simulink model "tau_11_1"  (R2019b)
settings: Solver=VariableStepAuto  StartTime=0.0  StopTime=1  RelTol=1e-3
libraries: simulink x16, slctrlblks x1
settings Model: PacingRate=0.001800  Creator=Sergey  LastModifiedBy=Sergey

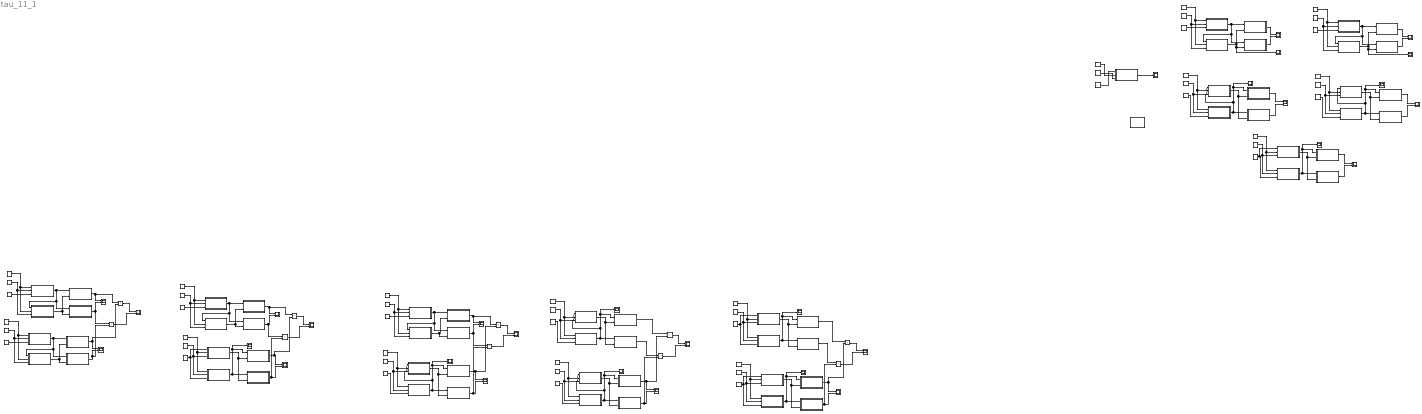
== system tau_11_1 ==
  note: А-ЗВЕНО
  note: П-ЗВЕНО
  note: РИ-ЗВЕНО
  note: ИИ-ЗВЕНО
  note: РД-ЗВЕНО
  note: А-ЗВЕНО
  note: А-ЗВЕНО
  note: А-ЗВЕНО
  note: РД-ЗВЕНО
  note: А-ЗВЕНО
  note: РИ-ЗВЕНО
  note: РИ-ЗВЕНО
  note: РИ-ЗВЕНО
  note: РД-ЗВЕНО
  note: РД-ЗВЕНО
  Bode Plot : slctrlblks/Model Verification/Check Bode  Characteristics  InstantiateOnLoad=on  SaveOperatingPoints=off  LinearizationIOs={}  LinearizeAt=SnapshotTimes  SnapshotTimes=[0]  TriggerType=rising  SampleTime=auto  RateConversionMethod=zoh  PreWarpFreq=10  UseExactDelayModel=off  UseFullBlockNameLabels=off  UseBusSignalLabels=off  enabled=on  stopWhenAssertionFail=off  export=off  ViewDlgPos=[1 41 1920 963]  OpenViewOnLoad=off  LaunchViewOnOpen=off  FrequencyUnits=rad/s  MagnitudeUnits=dB  PhaseUnits=deg  TimeUnits=seconds  EnableUpperBound=off  UpperBoundFrequencies=[]  UpperBoundMagnitudes=[]  EnableLowerBound=off  LowerBoundFrequencies=[]  LowerBoundMagnitudes=[]
      settings: SourceProductName=Simulink Control Design
  Constant{,4,8,10,12,14,16,18,20,22,24,26,28,30} (14 alike) : Constant  Value=0.5
  Constant{1,3,5,7,9,11,13,15,17,19,21,23,25,27,29,31} (16 alike) : Constant  Value=9
  Constant2 : Constant  Value=0
  Constant6 : Constant  Value=0
  MATLAB Function : MATLAB Function  TreatAsAtomicUnit=on
  MATLAB Function1 : MATLAB Function  TreatAsAtomicUnit=on
  MATLAB Function10 : MATLAB Function  TreatAsAtomicUnit=on
  MATLAB Function11 : MATLAB Function  TreatAsAtomicUnit=on
  MATLAB Function12 : MATLAB Function  TreatAsAtomicUnit=on
  MATLAB Function13 : MATLAB Function  TreatAsAtomicUnit=on
  MATLAB Function14 : MATLAB Function  TreatAsAtomicUnit=on
  MATLAB Function15 : MATLAB Function  TreatAsAtomicUnit=on
  MATLAB Function16 : MATLAB Function  TreatAsAtomicUnit=on
  MATLAB Function17 : MATLAB Function  TreatAsAtomicUnit=on
  MATLAB Function18 : MATLAB Function  TreatAsAtomicUnit=on
  MATLAB Function19 : MATLAB Function  TreatAsAtomicUnit=on
  MATLAB Function2 : MATLAB Function  TreatAsAtomicUnit=on
  MATLAB Function20 : MATLAB Function  TreatAsAtomicUnit=on
  MATLAB Function21 : MATLAB Function  TreatAsAtomicUnit=on
  MATLAB Function22 : MATLAB Function  TreatAsAtomicUnit=on
  MATLAB Function23 : MATLAB Function  TreatAsAtomicUnit=on
  MATLAB Function24 : MATLAB Function  TreatAsAtomicUnit=on
  MATLAB Function25 : MATLAB Function  TreatAsAtomicUnit=on
  MATLAB Function26 : MATLAB Function  TreatAsAtomicUnit=on
  MATLAB Function27 : MATLAB Function  TreatAsAtomicUnit=on
  MATLAB Function28 : MATLAB Function  TreatAsAtomicUnit=on
  MATLAB Function29 : MATLAB Function  TreatAsAtomicUnit=on
  MATLAB Function3 : MATLAB Function  TreatAsAtomicUnit=on
  MATLAB Function30 : MATLAB Function  TreatAsAtomicUnit=on
  MATLAB Function31 : MATLAB Function  TreatAsAtomicUnit=on
  MATLAB Function32 : MATLAB Function  TreatAsAtomicUnit=on
  MATLAB Function33 : MATLAB Function  TreatAsAtomicUnit=on
  MATLAB Function34 : MATLAB Function  TreatAsAtomicUnit=on
  MATLAB Function35 : MATLAB Function  TreatAsAtomicUnit=on
  MATLAB Function36 : MATLAB Function  TreatAsAtomicUnit=on
  MATLAB Function37 : MATLAB Function  TreatAsAtomicUnit=on
  MATLAB Function38 : MATLAB Function  TreatAsAtomicUnit=on
  MATLAB Function39 : MATLAB Function  TreatAsAtomicUnit=on
  MATLAB Function4 : MATLAB Function  TreatAsAtomicUnit=on
  MATLAB Function40 : MATLAB Function  TreatAsAtomicUnit=on
  MATLAB Function41 : MATLAB Function  TreatAsAtomicUnit=on
  MATLAB Function42 : MATLAB Function  TreatAsAtomicUnit=on
  MATLAB Function43 : MATLAB Function  TreatAsAtomicUnit=on
  MATLAB Function44 : MATLAB Function  TreatAsAtomicUnit=on
  MATLAB Function45 : MATLAB Function  TreatAsAtomicUnit=on
  MATLAB Function46 : MATLAB Function  TreatAsAtomicUnit=on
  MATLAB Function47 : MATLAB Function  TreatAsAtomicUnit=on
  MATLAB Function48 : MATLAB Function  TreatAsAtomicUnit=on
  MATLAB Function49 : MATLAB Function  TreatAsAtomicUnit=on
  MATLAB Function5 : MATLAB Function  TreatAsAtomicUnit=on
  MATLAB Function50 : MATLAB Function  TreatAsAtomicUnit=on
  MATLAB Function51 : MATLAB Function  TreatAsAtomicUnit=on
  MATLAB Function52 : MATLAB Function  TreatAsAtomicUnit=on
  MATLAB Function53 : MATLAB Function  TreatAsAtomicUnit=on
  MATLAB Function54 : MATLAB Function  TreatAsAtomicUnit=on
  MATLAB Function55 : MATLAB Function  TreatAsAtomicUnit=on
  MATLAB Function56 : MATLAB Function  TreatAsAtomicUnit=on
  MATLAB Function57 : MATLAB Function  TreatAsAtomicUnit=on
  MATLAB Function58 : MATLAB Function  TreatAsAtomicUnit=on
  MATLAB Function59 : MATLAB Function  TreatAsAtomicUnit=on
  MATLAB Function6 : MATLAB Function  TreatAsAtomicUnit=on
  MATLAB Function60 : MATLAB Function  TreatAsAtomicUnit=on
  MATLAB Function7 : MATLAB Function  TreatAsAtomicUnit=on
  MATLAB Function8 : MATLAB Function  TreatAsAtomicUnit=on
  MATLAB Function9 : MATLAB Function  TreatAsAtomicUnit=on
  Product{,1..9} (10 alike) : Product
  Ramp{,1..4,6..15} (15 alike) : simulink/Sources/Ramp  slope=1  start=0  InitialOutput=0
  Ramp5 : simulink/Sources/Ramp  slope=.0001  start=0  InitialOutput=0
  Scope{,2,4,6,8,11..17,19,21..22,25..26,28} (18 alike) : Scope  NumInputPorts=2
  Scope{1,3,5,7,9..10,18,20,23..24,27,29} (12 alike) : Scope
  wires:
  Ramp/1 -> MATLAB Function1/2(w), MATLAB Function/1(w)
  Constant/1 -> MATLAB Function1/3(T), MATLAB Function/2(T)
  Constant1/1 -> MATLAB Function/3(k)
  MATLAB Function/1(R) -> MATLAB Function3/1(R), MATLAB Function1/1(R), MATLAB Function2/1(R)
  MATLAB Function1/1(I) -> Scope1/1, MATLAB Function3/2(I), MATLAB Function2/2(I)
  MATLAB Function2/1(A) -> Scope/1
  MATLAB Function3/1(fi) -> Scope/2
  MATLAB Function7/1(fi) -> Scope2/2
  MATLAB Function6/1(A) -> Scope2/1
  MATLAB Function5/1(I) -> MATLAB Function6/2(I), MATLAB Function7/2(I), Scope3/1
  MATLAB Function4/1(R) -> MATLAB Function6/1(R), MATLAB Function5/1(R), MATLAB Function7/1(R)
  Constant3/1 -> MATLAB Function4/3(k)
  Constant2/1 -> MATLAB Function4/2(T), MATLAB Function5/3(T)
  Ramp1/1 -> MATLAB Function4/1(w), MATLAB Function5/2(w)
  MATLAB Function11/1(fi) -> Scope4/2
  MATLAB Function10/1(A) -> Scope4/1
  MATLAB Function9/1(R) -> MATLAB Function11/2(R), MATLAB Function10/2(R)
  MATLAB Function8/1(I) -> Scope5/1, MATLAB Function10/1(I), MATLAB Function9/3(I), MATLAB Function11/1(I)
  Constant5/1 -> MATLAB Function8/3(k)
  Constant4/1 -> MATLAB Function8/2(T), MATLAB Function9/2(T)
  Ramp2/1 -> MATLAB Function8/1(w), MATLAB Function9/1(w)
  Ramp3/1 -> MATLAB Function15/2(w), MATLAB Function14/1(w)
  Constant6/1 -> MATLAB Function15/3(T), MATLAB Function14/2(T)
  Constant7/1 -> MATLAB Function14/3(k)
  MATLAB Function14/1(I) -> MATLAB Function13/1(I), MATLAB Function15/1(I), MATLAB Function12/1(I), Scope7/1
  MATLAB Function15/1(R) -> MATLAB Function12/2(R), MATLAB Function13/2(R)
  MATLAB Function12/1(A) -> Scope6/1
  MATLAB Function13/1(fi) -> Scope6/2
  Ramp4/1 -> MATLAB Function19/2(w), MATLAB Function18/1(w)
  Constant8/1 -> MATLAB Function19/3(T), MATLAB Function18/2(T)
  Constant9/1 -> MATLAB Function19/1(k), MATLAB Function18/3(k)
  MATLAB Function18/1(I) -> MATLAB Function17/1(I), MATLAB Function16/1(I), Scope9/1
  MATLAB Function19/1(R) -> MATLAB Function16/2(R), MATLAB Function17/2(R)
  MATLAB Function16/1(A) -> Scope8/1
  MATLAB Function17/1(fi) -> Scope8/2
  Constant11/1 -> MATLAB Function20/1(k)
  Constant10/1 -> MATLAB Function20/3(T)
  MATLAB Function20/1(R) -> Scope10/1
  Ramp5/1 -> MATLAB Function20/2(w)
  MATLAB Function24/1(fi) -> Product/1, Scope11/2
  MATLAB Function23/1(A) -> Product1/1, Scope11/1
  MATLAB Function22/1(I) -> MATLAB Function23/2(I), MATLAB Function24/2(I)
  MATLAB Function21/1(R) -> MATLAB Function23/1(R), MATLAB Function22/1(R), MATLAB Function24/1(R)
  Constant13/1 -> MATLAB Function21/3(k)
  Constant12/1 -> MATLAB Function21/2(T), MATLAB Function22/3(T)
  Ramp6/1 -> MATLAB Function21/1(w), MATLAB Function22/2(w)
  Ramp7/1 -> MATLAB Function26/2(w), MATLAB Function25/1(w)
  Constant14/1 -> MATLAB Function26/3(T), MATLAB Function25/2(T)
  Constant15/1 -> MATLAB Function25/3(k)
  MATLAB Function25/1(R) -> MATLAB Function28/1(R), MATLAB Function26/1(R), MATLAB Function27/1(R)
  MATLAB Function26/1(I) -> MATLAB Function28/2(I), MATLAB Function27/2(I)
  MATLAB Function27/1(A) -> Product1/2, Scope12/1
  MATLAB Function28/1(fi) -> Product/2, Scope12/2
  Product1/1 -> Scope13/1
  Product/1 -> Scope13/2
  Product2/1 -> Scope16/2
  Product3/1 -> Scope16/1
  Ramp8/1 -> MATLAB Function30/2(w), MATLAB Function29/1(w)
  Constant16/1 -> MATLAB Function30/3(T), MATLAB Function29/2(T)
  Constant17/1 -> MATLAB Function29/3(k)
  MATLAB Function29/1(R) -> MATLAB Function32/1(R), MATLAB Function30/1(R), MATLAB Function31/1(R)
  MATLAB Function30/1(I) -> MATLAB Function32/2(I), MATLAB Function31/2(I)
  MATLAB Function31/1(A) -> Scope14/1, Product3/1
  MATLAB Function32/1(fi) -> Scope14/2, Product2/1
  MATLAB Function38/1(fi) -> Product2/2, Scope17/2
  MATLAB Function37/1(A) -> Product3/2, Scope17/1
  MATLAB Function40/1(R) -> MATLAB Function38/2(R), MATLAB Function37/2(R)
  MATLAB Function39/1(I) -> Scope18/1, MATLAB Function37/1(I), MATLAB Function38/1(I)
  Constant21/1 -> MATLAB Function39/3(k), MATLAB Function40/1(k)
  Constant20/1 -> MATLAB Function39/2(T), MATLAB Function40/3(T)
  Ramp10/1 -> MATLAB Function39/1(w), MATLAB Function40/2(w)
  MATLAB Function36/1(fi) -> Product4/1, Scope15/2
  MATLAB Function35/1(A) -> Product5/1, Scope15/1
  MATLAB Function34/1(I) -> MATLAB Function35/2(I), MATLAB Function36/2(I)
  MATLAB Function33/1(R) -> MATLAB Function35/1(R), MATLAB Function34/1(R), MATLAB Function36/1(R)
  Constant19/1 -> MATLAB Function33/3(k)
  Constant18/1 -> MATLAB Function33/2(T), MATLAB Function34/3(T)
  Ramp11/1 -> MATLAB Function33/1(w), MATLAB Function34/2(w)
  Product5/1 -> Scope19/1
  Product4/1 -> Scope19/2
  Ramp14/1 -> MATLAB Function56/1(w), MATLAB Function55/1(w)
  Constant28/1 -> MATLAB Function56/2(T), MATLAB Function55/2(T)
  Constant29/1 -> MATLAB Function55/3(k)
  MATLAB Function55/1(I) -> MATLAB Function54/1(I), MATLAB Function56/3(I), MATLAB Function53/1(I), Scope27/1
  MATLAB Function56/1(R) -> MATLAB Function53/2(R), MATLAB Function54/2(R)
  MATLAB Function53/1(A) -> Product5/2, Scope26/1
  MATLAB Function54/1(fi) -> Product4/2, Scope26/2
  MATLAB Function46/1(fi) -> Scope22/2, Product6/2
  MATLAB Function45/1(A) -> Scope22/1, Product7/2
  MATLAB Function48/1(R) -> MATLAB Function46/2(R), MATLAB Function45/2(R)
  MATLAB Function47/1(I) -> Scope23/1, MATLAB Function45/1(I), MATLAB Function48/3(I), MATLAB Function46/1(I)
  Constant25/1 -> MATLAB Function47/3(k)
  Constant24/1 -> MATLAB Function47/2(T), MATLAB Function48/2(T)
  Ramp12/1 -> MATLAB Function47/1(w), MATLAB Function48/1(w)
  Product6/1 -> Scope21/2
  Product7/1 -> Scope21/1
  Ramp9/1 -> MATLAB Function44/1(w), MATLAB Function43/1(w)
  Constant22/1 -> MATLAB Function44/2(T), MATLAB Function43/2(T)
  Constant23/1 -> MATLAB Function43/3(k)
  MATLAB Function43/1(I) -> MATLAB Function42/1(I), MATLAB Function44/3(I), MATLAB Function41/1(I), Scope20/1
  MATLAB Function44/1(R) -> MATLAB Function41/2(R), MATLAB Function42/2(R)
  MATLAB Function42/1(fi) -> Product6/1
  MATLAB Function41/1(A) -> Product7/1
  Ramp13/1 -> MATLAB Function60/2(w), MATLAB Function59/1(w)
  Constant30/1 -> MATLAB Function60/3(T), MATLAB Function59/2(T)
  Constant31/1 -> MATLAB Function60/1(k), MATLAB Function59/3(k)
  MATLAB Function59/1(I) -> MATLAB Function58/1(I), MATLAB Function57/1(I), Scope29/1
  MATLAB Function60/1(R) -> MATLAB Function57/2(R), MATLAB Function58/2(R)
  MATLAB Function57/1(A) -> Scope28/1, Product9/2
  MATLAB Function58/1(fi) -> Scope28/2, Product8/2
  Product9/1 -> Scope25/1
  Product8/1 -> Scope25/2
  MATLAB Function52/1(R) -> MATLAB Function50/2(R), MATLAB Function49/2(R)
  MATLAB Function51/1(I) -> Scope24/1, MATLAB Function49/1(I), MATLAB Function50/1(I)
  Constant27/1 -> MATLAB Function51/3(k), MATLAB Function52/1(k)
  Constant26/1 -> MATLAB Function51/2(T), MATLAB Function52/3(T)
  Ramp15/1 -> MATLAB Function51/1(w), MATLAB Function52/2(w)
  MATLAB Function50/1(fi) -> Product8/1
  MATLAB Function49/1(A) -> Product9/1

== matlab function tau_11_1/MATLAB Function1 ==
  data: R input; w input; I output; T input
function I = fcn(R,w,T)

I = R*w*T;
I = -I;

== matlab function tau_11_1/MATLAB Function ==
  data: w input; R output; T input; k input
function R = fcn(w,T,k)

R = k/(1+w^2*T^2);

== matlab function tau_11_1/MATLAB Function2 ==
  data: R input; I input; A output
function A = fcn(R,I)

A = R^2+I^2;
A = sqrt(A);

== matlab function tau_11_1/MATLAB Function3 ==
  data: R input; I input; fi output
function fi = fcn(R,I)


fi = atan2(I,R);

== matlab function tau_11_1/MATLAB Function4 ==
  data: w input; R output; T input; k input
function R = fcn(w,T,k)

R = k/(1+w^2*T^2);

== matlab function tau_11_1/MATLAB Function5 ==
  data: R input; w input; I output; T input
function I = fcn(R,w,T)

I = R*w*T;
I = -I;

== matlab function tau_11_1/MATLAB Function6 ==
  data: R input; I input; A output
function A = fcn(R,I)

A = R^2+I^2;
A = sqrt(A);

== matlab function tau_11_1/MATLAB Function7 ==
  data: R input; I input; fi output
function fi = fcn(R,I)


fi = atan2(I,R);

== matlab function tau_11_1/MATLAB Function10 ==
  data: I input; R input; A output
function A = fcn(I,R)

A = R^2+I^2;
A = sqrt(A);

== matlab function tau_11_1/MATLAB Function11 ==
  data: I input; R input; fi output
function fi = fcn(I,R)


fi = atan2(I,R);

== matlab function tau_11_1/MATLAB Function8 ==
  data: w input; I output; T input; k input
function I = fcn(w,T,k)

I = k/(w*(1+w^2*T^2));
I = -I;

== matlab function tau_11_1/MATLAB Function9 ==
  data: w input; T input; I input; R output
function R = fcn(w,T,I)


R = I*w*T;

== matlab function tau_11_1/MATLAB Function12 ==
  data: I input; R input; A output
function A = fcn(I,R)

A = R^2+I^2;
A = sqrt(A);

== matlab function tau_11_1/MATLAB Function13 ==
  data: I input; R input; fi output
function fi = fcn(I,R)


fi = atan2(I,R);

== matlab function tau_11_1/MATLAB Function14 ==
  data: w input; I output; T input; k input
function I = fcn(w,T,k)

I = k/(w*(1+w^2*T^2));
I = -I;

== matlab function tau_11_1/MATLAB Function15 ==
  data: I input; w input; R output; T input
function R = fcn(I,w,T)


R = I*w*T;

== matlab function tau_11_1/MATLAB Function16 ==
  data: I input; R input; A output
function A = fcn(I,R)

A = R^2+I^2;
A = sqrt(A);

== matlab function tau_11_1/MATLAB Function17 ==
  data: I input; R input; fi output
function fi = fcn(I,R)


fi = atan2(I,R);

== matlab function tau_11_1/MATLAB Function18 ==
  data: w input; I output; T input; k input
function I = fcn(w,T,k)

I = (k*w)/(1+w^2*T^2);

== matlab function tau_11_1/MATLAB Function19 ==
  data: k input; w input; R output; T input
function R = fcn(k,w,T)


R = (w^2*T*k)/(1+w^2*T^2);

== matlab function tau_11_1/MATLAB Function20 ==
  data: k input; w input; T input; R output
function R = fcn(k,w,T)


R = k/(w*sqrt(1+w^2*T^2));

== matlab function tau_11_1/MATLAB Function21 ==
  data: w input; R output; T input; k input
function R = fcn(w,T,k)

R = k/(1+w^2*T^2);

== matlab function tau_11_1/MATLAB Function22 ==
  data: R input; w input; I output; T input
function I = fcn(R,w,T)

I = R*w*T;
I = -I;

== matlab function tau_11_1/MATLAB Function23 ==
  data: R input; I input; A output
function A = fcn(R,I)

A = R^2+I^2;
A = sqrt(A);

== matlab function tau_11_1/MATLAB Function24 ==
  data: R input; I input; fi output
function fi = fcn(R,I)


fi = atan2(I,R);

== matlab function tau_11_1/MATLAB Function25 ==
  data: w input; R output; T input; k input
function R = fcn(w,T,k)

R = k/(1+w^2*T^2);

== matlab function tau_11_1/MATLAB Function26 ==
  data: R input; w input; I output; T input
function I = fcn(R,w,T)

I = R*w*T;
I = -I;

== matlab function tau_11_1/MATLAB Function27 ==
  data: R input; I input; A output
function A = fcn(R,I)

A = R^2+I^2;
A = sqrt(A);

== matlab function tau_11_1/MATLAB Function28 ==
  data: R input; I input; fi output
function fi = fcn(R,I)


fi = atan2(I,R);

== matlab function tau_11_1/MATLAB Function29 ==
  data: w input; R output; T input; k input
function R = fcn(w,T,k)

R = k/(1+w^2*T^2);

== matlab function tau_11_1/MATLAB Function30 ==
  data: R input; w input; I output; T input
function I = fcn(R,w,T)

I = R*w*T;
I = -I;

== matlab function tau_11_1/MATLAB Function31 ==
  data: R input; I input; A output
function A = fcn(R,I)

A = R^2+I^2;
A = sqrt(A);

== matlab function tau_11_1/MATLAB Function32 ==
  data: R input; I input; fi output
function fi = fcn(R,I)


fi = atan2(I,R);

== matlab function tau_11_1/MATLAB Function33 ==
  data: w input; R output; T input; k input
function R = fcn(w,T,k)

R = k/(1+w^2*T^2);

== matlab function tau_11_1/MATLAB Function34 ==
  data: R input; w input; I output; T input
function I = fcn(R,w,T)

I = R*w*T;
I = -I;

== matlab function tau_11_1/MATLAB Function35 ==
  data: R input; I input; A output
function A = fcn(R,I)

A = R^2+I^2;
A = sqrt(A);

== matlab function tau_11_1/MATLAB Function36 ==
  data: R input; I input; fi output
function fi = fcn(R,I)


fi = atan2(I,R);

== matlab function tau_11_1/MATLAB Function37 ==
  data: I input; R input; A output
function A = fcn(I,R)

A = R^2+I^2;
A = sqrt(A);

== matlab function tau_11_1/MATLAB Function38 ==
  data: I input; R input; fi output
function fi = fcn(I,R)


fi = atan2(I,R);

== matlab function tau_11_1/MATLAB Function39 ==
  data: w input; I output; T input; k input
function I = fcn(w,T,k)

I = (k*w)/(1+w^2*T^2);

== matlab function tau_11_1/MATLAB Function40 ==
  data: k input; w input; R output; T input
function R = fcn(k,w,T)


R = (w^2*T*k)/(1+w^2*T^2);

== matlab function tau_11_1/MATLAB Function41 ==
  data: I input; R input; A output
function A = fcn(I,R)

A = R^2+I^2;
A = sqrt(A);

== matlab function tau_11_1/MATLAB Function42 ==
  data: I input; R input; fi output
function fi = fcn(I,R)


fi = atan2(I,R);

== matlab function tau_11_1/MATLAB Function43 ==
  data: w input; I output; T input; k input
function I = fcn(w,T,k)

I = k/(w*(1+w^2*T^2));
I = -I;

== matlab function tau_11_1/MATLAB Function44 ==
  data: w input; T input; I input; R output
function R = fcn(w,T,I)


R = I*w*T;

== matlab function tau_11_1/MATLAB Function45 ==
  data: I input; R input; A output
function A = fcn(I,R)

A = R^2+I^2;
A = sqrt(A);

== matlab function tau_11_1/MATLAB Function46 ==
  data: I input; R input; fi output
function fi = fcn(I,R)


fi = atan2(I,R);

== matlab function tau_11_1/MATLAB Function47 ==
  data: w input; I output; T input; k input
function I = fcn(w,T,k)

I = k/(w*(1+w^2*T^2));
I = -I;

== matlab function tau_11_1/MATLAB Function48 ==
  data: w input; T input; I input; R output
function R = fcn(w,T,I)


R = I*w*T;

== matlab function tau_11_1/MATLAB Function49 ==
  data: I input; R input; A output
function A = fcn(I,R)

A = R^2+I^2;
A = sqrt(A);

== matlab function tau_11_1/MATLAB Function50 ==
  data: I input; R input; fi output
function fi = fcn(I,R)


fi = atan2(I,R);

== matlab function tau_11_1/MATLAB Function51 ==
  data: w input; I output; T input; k input
function I = fcn(w,T,k)

I = (k*w)/(1+w^2*T^2);

== matlab function tau_11_1/MATLAB Function52 ==
  data: k input; w input; R output; T input
function R = fcn(k,w,T)


R = (w^2*T*k)/(1+w^2*T^2);

== matlab function tau_11_1/MATLAB Function53 ==
  data: I input; R input; A output
function A = fcn(I,R)

A = R^2+I^2;
A = sqrt(A);

== matlab function tau_11_1/MATLAB Function54 ==
  data: I input; R input; fi output
function fi = fcn(I,R)


fi = atan2(I,R);

== matlab function tau_11_1/MATLAB Function55 ==
  data: w input; I output; T input; k input
function I = fcn(w,T,k)

I = k/(w*(1+w^2*T^2));
I = -I;

== matlab function tau_11_1/MATLAB Function56 ==
  data: w input; T input; I input; R output
function R = fcn(w,T,I)


R = I*w*T;

== matlab function tau_11_1/MATLAB Function57 ==
  data: I input; R input; A output
function A = fcn(I,R)

A = R^2+I^2;
A = sqrt(A);

== matlab function tau_11_1/MATLAB Function58 ==
  data: I input; R input; fi output
function fi = fcn(I,R)


fi = atan2(I,R);

== matlab function tau_11_1/MATLAB Function59 ==
  data: w input; I output; T input; k input
function I = fcn(w,T,k)

I = (k*w)/(1+w^2*T^2);

== matlab function tau_11_1/MATLAB Function60 ==
  data: k input; w input; R output; T input
function R = fcn(k,w,T)


R = (w^2*T*k)/(1+w^2*T^2);
